simulink model "DiagramaParaTexto"  (Simulink 7.7)
settings: Solver=ode45  StartTime=0.0  StopTime=300  RelTol=1e-3
undefined symbols (not defined in the file or in its folder): analoginput, analogoutput, C1, C2, D12, D21, QT, u1_Estacionario, u2_Estacionario
libraries: daqlib x2
settings Model: Creator=didaticontrol  LastModifiedBy=Arthur
settings OptimizationCC: InitFltsAndDblsToZero=on
settings DebuggingCC: StrictBusMsg=Warning

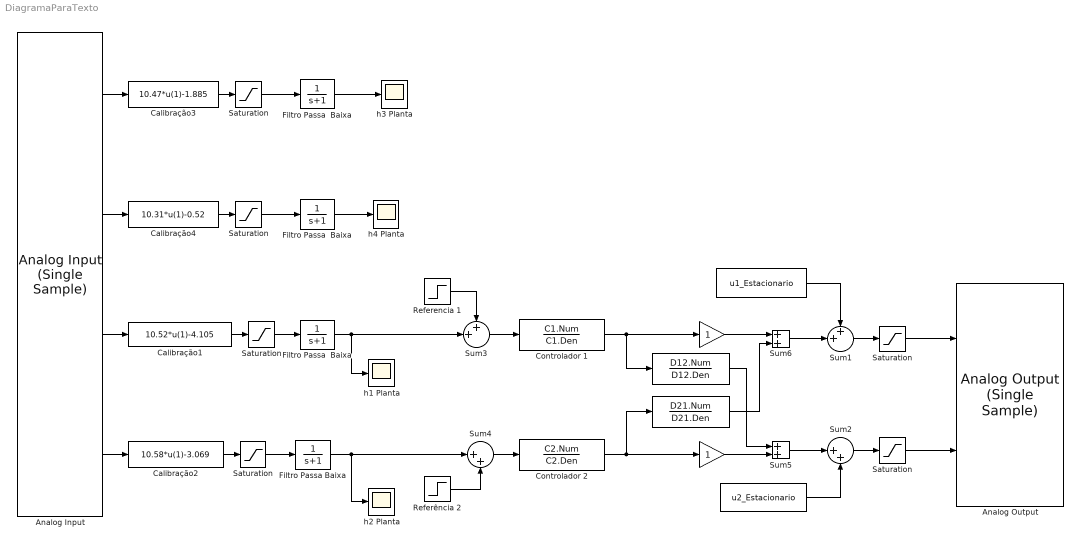
== system DiagramaParaTexto ==
  " " : Gain
  "  " : Gain
  "   " : TransferFcn  Numerator=D12.Num  Denominator=D12.Den
  "    " : TransferFcn  Numerator=D21.Num  Denominator=D21.Den
  "     " : Constant  Value=u1_Estacionario
  "      " : Constant  Value=u2_Estacionario
  Analog Input : daqlib/Analog Input (Single Sample)  DeviceMenu=nidaq Dev1 (USB-6008)  Device=nidaq Dev1 (USB-6008)  ObjConstructor=analoginput('nidaq','Dev1')  InputType=Differential  NChannelsSelected=4  Channels=1$0$$5$#1$1$$5$#1$2$$5$#1$3$$5$#  NPorts=1 per hardware channel  BlockSampleTime=10e-3
  Analog Output : daqlib/Analog Output (Single Sample)  DeviceMenu=nidaq Dev1 (USB-6008)  Device=nidaq Dev1 (USB-6008)  ObjConstructor=analogoutput('nidaq','Dev1')  NChannelsSelected=2  Channels=1$0$$1$0$#1$1$$1$0$#  NPorts=1 per hardware channel
  Calibração1 : Fcn  Expr=10.52*u(1)-4.105  SampleTime=10e-3
  Calibração2 : Fcn  Expr=10.58*u(1)-3.069
  Calibração3 : Fcn  Expr=10.47*u(1)-1.885
  Calibração4 : Fcn  Expr=10.31*u(1)-0.52
  Controlador 1 : TransferFcn  Numerator=C1.Num  Denominator=C1.Den
  Controlador 2 : TransferFcn  Numerator=C2.Num  Denominator=C2.Den
  Filtro Passa  Baixa : TransferFcn  Denominator=[1 1]
  "Filtro Passa  Baixa " : TransferFcn  Denominator=[1 1]
  "Filtro Passa  Baixa  " : TransferFcn  Denominator=[1 1]
  "Filtro Passa Baixa   " : TransferFcn  Denominator=[1 1]
  Referencia 1 : Step  Time=100  Before=QT.ctes.h0(1)  After=QT.ctes.h0(1)+1
  Referência 2 : Step  Time=200  Before=QT.ctes.h0(2)  After=QT.ctes.h0(2)+1  SampleTime=0
  "Saturation " : Saturate  UpperLimit=23  LowerLimit=0
  "Saturation  " : Saturate  UpperLimit=23  LowerLimit=0
  "Saturation   " : Saturate  UpperLimit=23  LowerLimit=0  SampleTime=10e-3
  "Saturation    " : Saturate  UpperLimit=23  LowerLimit=0
  "Saturation       " : Saturate  UpperLimit=0.7*5  LowerLimit=0  SampleTime=10e-3
  "Saturation        " : Saturate  UpperLimit=0.7*5  LowerLimit=0  SampleTime=10e-3
  Sum1 : Sum  Inputs=++|
  Sum2 : Sum  Inputs=|++
  Sum3 : Sum  Inputs=++|
  Sum4 : Sum  Inputs=|++
  Sum5 : Sum
  Sum6 : Sum
  h1 Planta : Scope
      settings: TimeRange=300  YMin=0  YMax=9  SaveName=h1_real  SampleInput=on  SampleTime=10e-3
  h2 Planta : Scope
      settings: TimeRange=300  YMin=0  YMax=9.5  SaveName=h2_real  SampleInput=on  SampleTime=10e-3
  h3 Planta : Scope
      settings: TimeRange=300  YMin=0  YMax=10.5  SaveName=h3_real  SampleInput=on  SampleTime=10e-3
  h4 Planta : Scope
      settings: YMin=0  YMax=12  SaveName=h4_real  SampleInput=on  SampleTime=10e-3
  wires:
  Analog Input/3 -> Calibração1/1
  Calibração1/1 -> "Saturation   "/1
  Calibração2/1 -> "Saturation    "/1
  Analog Input/4 -> Calibração2/1
  Analog Input/2 -> Calibração4/1
  Analog Input/1 -> Calibração3/1
  Calibração3/1 -> "Saturation "/1
  Calibração4/1 -> "Saturation  "/1
  "Saturation        "/1 -> Analog Output/2
  Referência 2/1 -> Sum4/2
  Sum1/1 -> "Saturation       "/1
  Sum2/1 -> "Saturation        "/1
  "Saturation       "/1 -> Analog Output/1
  "Saturation "/1 -> Filtro Passa  Baixa/1
  "Saturation  "/1 -> "Filtro Passa  Baixa "/1
  "Filtro Passa  Baixa  "/1 -> h1 Planta/1, Sum3/2
  "Saturation   "/1 -> "Filtro Passa  Baixa  "/1
  "Saturation    "/1 -> "Filtro Passa Baixa   "/1
  "Filtro Passa  Baixa "/1 -> h4 Planta/1
  Filtro Passa  Baixa/1 -> h3 Planta/1
  Referencia 1/1 -> Sum3/1
  "      "/1 -> Sum2/2
  "Filtro Passa Baixa   "/1 -> Sum4/1, h2 Planta/1
  "     "/1 -> Sum1/1
  Sum6/1 -> Sum1/2
  "    "/1 -> Sum6/2
  Sum5/1 -> Sum2/1
  "   "/1 -> Sum5/1
  "  "/1 -> Sum5/2
  " "/1 -> Sum6/1
  Controlador 1/1 -> "   "/1, " "/1
  Controlador 2/1 -> "    "/1, "  "/1
  Sum3/1 -> Controlador 1/1
  Sum4/1 -> Controlador 2/1
